simulink model "intes_cross_2018b_acc"  (R2018b)
settings: Solver=VariableStepAuto  StartTime=0.0  StopTime=10.0  RelTol=1e-3
settings Model: Creator=lenovo  LastModifiedBy=lenovo

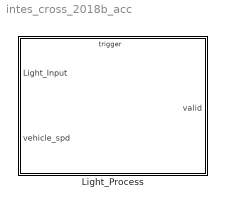
== system intes_cross_2018b_acc ==
  Light_Process : Subsystem

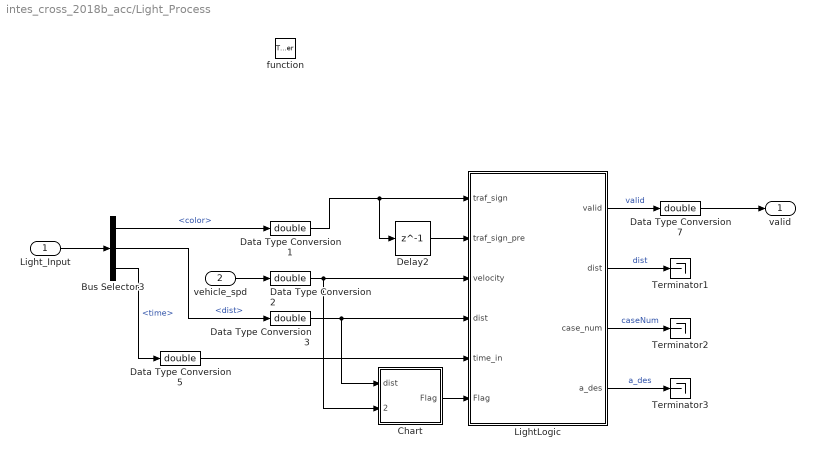
== system intes_cross_2018b_acc/Light_Process ==
  Light_Input : Inport  OutDataTypeStr=Bus: Light_Info_ST  BusOutputAsStruct=on
  vehicle_spd : Inport  Port=2  BusOutputAsStruct=on
  function : TriggerPort  TriggerType=function-call  VariantControl=Variant
  Bus Selector3 : BusSelector  OutputSignals=color,dist,time
  Chart : Stateflow chart  TreatAsAtomicUnit=on
  Data Type Conversion{1..3,5,7} (5 alike) : DataTypeConversion  OutDataTypeStr=double
  Delay2 : Delay  DelayLength=1
  LightLogic : MATLAB Function  TreatAsAtomicUnit=on
  Terminator1 : Terminator
  Terminator2 : Terminator
  Terminator3 : Terminator
  valid : Outport
  wires:
  Data Type Conversion7/1 -> valid/1
  Light_Input/1 -> Bus Selector3/1
  Bus Selector3/1 -> Data Type Conversion1/1  "<color>"
  Bus Selector3/2 -> Data Type Conversion3/1  "<dist>"
  vehicle_spd/1 -> Data Type Conversion2/1
  Bus Selector3/3 -> Data Type Conversion5/1  "<time>"
  Data Type Conversion1/1 -> LightLogic/1(traf_sign), Delay2/1
  Data Type Conversion3/1 -> LightLogic/4("dist "), Chart/1(dist)
  Data Type Conversion5/1 -> LightLogic/5(time_in)
  Data Type Conversion2/1 -> LightLogic/3(velocity), Chart/2(velocity)
  LightLogic/2(dist) -> Terminator1/1  "dist"
  Chart/1(Flag) -> LightLogic/6(Flag)
  LightLogic/1(valid) -> Data Type Conversion7/1  "valid"
  Delay2/1 -> LightLogic/2(traf_sign_pre)
  LightLogic/3(case_num) -> Terminator2/1  "caseNum"
  LightLogic/4(a_des) -> Terminator3/1  "a_des"

== stateflow chart intes_cross_2018b_acc/Light_Process/Chart ==
  state init
    en:
    Flag=0;
  state Off
    en:
    Flag=0;
  state On
    du:
    Flag=1;
  (default) -> init
  init -> On : [dist > 0 && dist / (velocity + 0.0001) <= 5]
  Off -> init : [dist > 0]
  On -> Off : [dist < -5]
  data: dist input; velocity input; Flag output

== matlab function intes_cross_2018b_acc/Light_Process/LightLogic ==
  data: valid output; traf_sign input; traf_sign_pre input; velocity input; dist input; time_in input; dist output; case_num output; Flag input; a_des output
function [ valid,dist,case_num,a_des] = intesec_cross( traf_sign,traf_sign_pre, velocity, dist, time_in, Flag)  
%% this is a function that provide desired velocity, and distance to traffic light;
    % input: trafic_sign with green = 0; red = 1; yellow = 2;
    %        velocity in unit of kph;
    %        dist, and time is distance(m) to cross, and traffic time left
    %        CONST_LIMIT is velocity limit at cross, which is a reference CONSTANT velocity from
    %        ACC module.
    %        v_des_pre preseve previous v_des for next step use.
    
    % output: desired velocity for ACC module, in unit of kph;
    %         dist is distance(m) to front cross;
   
    case_num = 0;
    time = time_in;
    green = 1;
    red = 3;
    yellow = 2;
    v = velocity;
%     if time == 2
%         a_des = 0;
%          v_des = 0;
%     end
    
    if (Flag == 0)
       
        a_des = 0;
        dist = 100;
        case_num = 0;
        valid = 0;
        
        return;
    end
    
    if dist < 0
        if traf_sign == green
            dist = 200;
        else
            dist = 0;
        end
    end
    
    if (Flag == 1)

        
        % CONST_LIMIT = CONST_LIMIT;
        
        ttc = dist / (v + 0.001);
        ttc = max(0,ttc);

        if traf_sign == green
            time = time + 3;
        elseif traf_sign == yellow
            traf_sign = green;
        end

        switch traf_sign
            case green
                if time < 7
                    valid = 1;
                    case_num = 1;
                elseif (ttc > time && v > 0.5)
                    valid = 1;
                    case_num = 2;
                   
                else
                    valid = 0;
                    case_num = 3;
                end

            case red
                valid = 1;
                case_num = 4;
            otherwise
                valid = 0;
                case_num = 5;
        end
        
    else
                valid = 0;
         
    end
    
    if valid == 1
        a_des = v^2 / (2 * dist);
    else 
        a_des = 1;
    end
   
end
